simulink model "Waermepumpe"  (R2013a)
settings: Solver=ode45  StartTime=0.0  StopTime=1000  RelTol=1e-3
libraries: Thermolib x21
settings Model: Creator=admin  LastModifiedBy=studi

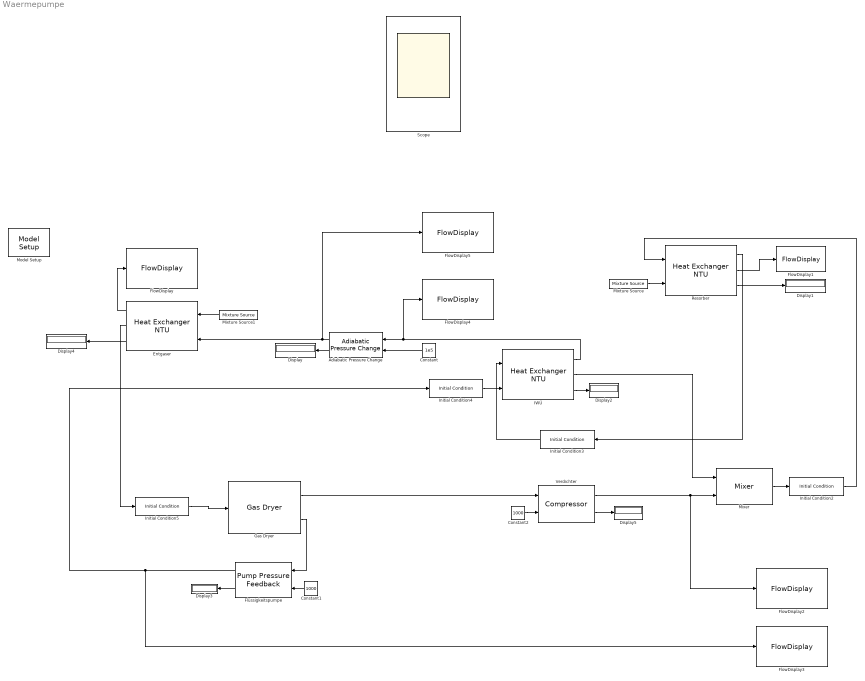
== system Waermepumpe ==
  Adiabatic Pressure Change : Thermolib/Thermodynamic State Changes/Adiabatic Pressure Change
  Constant : Constant  Value=1e5
  Constant1 : Constant  Value=1000
  Constant2 : Constant  Value=1000
  Display{,1..5} (6 alike) : Display
  Entgaser : Thermolib/Components/Heat and Mass Transfer/Heat Exchanger NTU  selection=Counter Flow  show_UA_port=off  UA_Overall=1e3  T_initial=273+25  A_env=1  T_env=273+25  k_env=0  p_loss_1=[0,1e3]  p_loss_2=[0,1e3]  thermal_mass=1*4.18e3  UA_flow1_mass1=0  UA_flow2_mass2=0  show_pf_ports=off  show_info_port=off  default_order_in_ports={'in1','in2','PFin1','PFin2'}  default_order_out_ports={'out1','out2','Qdot','PFout1','PFout2','info'}
  FlowDisplay : Thermolib/Sinks/FlowDisplay  bus_type=FlowBus  mdot=off kg/s  m_unit=mg  ndot=on mol/s  n_unit=mmol  temperature=on  T_unit=Kelvin  pressure=on  p_unit=Pa  enthalpy=off  Hdot_unit=W  H_unit=mJ  entropy=off  Sdot_unit=W/K  S_unit=mJ/K  gibbs_energy=off  Gdot_unit=W  G_unit=mJ  heat_capacity=on  Cpdot_unit=W/K  Cp_unit=mJ/K  energy_content=off  U_unit=mW/K  vapor_fraction=off  molar_fraction=off  flag=0.0921
  FlowDisplay1 : Thermolib/Sinks/FlowDisplay  bus_type=FlowBus  mdot=off kg/s  m_unit=mg  ndot=on mol/s  n_unit=mmol  temperature=on  T_unit=Kelvin  pressure=on  p_unit=Pa  enthalpy=on  Hdot_unit=W  H_unit=mJ  entropy=off  Sdot_unit=W/K  S_unit=mJ/K  gibbs_energy=off  Gdot_unit=W  G_unit=mJ  heat_capacity=off  Cpdot_unit=W/K  Cp_unit=mJ/K  energy_content=off  U_unit=mW/K  vapor_fraction=off  molar_fraction=off  flag=0.1161
  FlowDisplay2 : Thermolib/Sinks/FlowDisplay  bus_type=FlowBus  mdot=off kg/s  m_unit=mg  ndot=on mol/s  n_unit=mmol  temperature=on  T_unit=Kelvin  pressure=on  p_unit=bar  enthalpy=off  Hdot_unit=W  H_unit=mJ  entropy=off  Sdot_unit=W/K  S_unit=mJ/K  gibbs_energy=off  Gdot_unit=W  G_unit=mJ  heat_capacity=on  Cpdot_unit=W/K  Cp_unit=mJ/K  energy_content=off  U_unit=mW/K  vapor_fraction=off  molar_fraction=off  flag=0.4963
  FlowDisplay3 : Thermolib/Sinks/FlowDisplay  bus_type=FlowBus  mdot=off kg/s  m_unit=mg  ndot=on mol/s  n_unit=mmol  temperature=on  T_unit=Kelvin  pressure=on  p_unit=bar  enthalpy=off  Hdot_unit=W  H_unit=mJ  entropy=off  Sdot_unit=W/K  S_unit=mJ/K  gibbs_energy=off  Gdot_unit=W  G_unit=mJ  heat_capacity=on  Cpdot_unit=W/K  Cp_unit=mJ/K  energy_content=off  U_unit=mW/K  vapor_fraction=off  molar_fraction=off  flag=0.3209
  FlowDisplay4 : Thermolib/Sinks/FlowDisplay  bus_type=FlowBus  mdot=off kg/s  m_unit=mg  ndot=on mol/s  n_unit=mmol  temperature=on  T_unit=Kelvin  pressure=on  p_unit=bar  enthalpy=off  Hdot_unit=W  H_unit=mJ  entropy=off  Sdot_unit=W/K  S_unit=mJ/K  gibbs_energy=off  Gdot_unit=W  G_unit=mJ  heat_capacity=on  Cpdot_unit=W/K  Cp_unit=mJ/K  energy_content=off  U_unit=mW/K  vapor_fraction=off  molar_fraction=off  flag=0.5847
  FlowDisplay5 : Thermolib/Sinks/FlowDisplay  bus_type=FlowBus  mdot=off kg/s  m_unit=mg  ndot=on mol/s  n_unit=mmol  temperature=on  T_unit=Kelvin  pressure=on  p_unit=bar  enthalpy=off  Hdot_unit=W  H_unit=mJ  entropy=off  Sdot_unit=W/K  S_unit=mJ/K  gibbs_energy=off  Gdot_unit=W  G_unit=mJ  heat_capacity=on  Cpdot_unit=W/K  Cp_unit=mJ/K  energy_content=off  U_unit=mW/K  vapor_fraction=off  molar_fraction=off  flag=0.7896
  Flüssigkeitspumpe : Thermolib/Components/Hydraulic with Pressure Feedback/Pump Pressure Feedback  Mode=feed  eta_pump="[0.0 1.0;  0.8  0.8]"  RPM=[0 3000 4000 5000]  mdot=[0 8 16 24 32 34]*1e6/3600  PressureRise=[0 0 0 0 0 0 ; 13 12 10.7 8.3 3 0 ; 13 12 10.7 8.3 3 0; 13 12 10.7 8.3 3 0]*9.81e3  max_mdot=34e6/3600  p_refrence=2e5  p_Relaxation=10  show_pf_ports=off  show_info_port=off  default_order_in_ports={'in','RPM','PFin'}  default_order_out_ports={'out','P_mch','PFout','info'}
  Gas Dryer : Thermolib/Components/Heat and Mass Transfer/Gas Dryer  Abscheid_eff=[1 1 1 1 1]  ndots=[0 0.05 0.2 1 1.1]  P_Loss=[0.0,1e3]  show_pf_ports=off  show_info_port=off  default_order_in_ports={'in','PFin'}  default_order_out_ports={'out','liquid','PFout','info'}
  IWÜ : Thermolib/Components/Heat and Mass Transfer/Heat Exchanger NTU  selection=Counter Flow  show_UA_port=off  UA_Overall=1e3  T_initial=273+25  A_env=1  T_env=273+20  k_env=0  p_loss_1=[0,1e3]  p_loss_2=[0,1e3]  thermal_mass=1*4.18e3  UA_flow1_mass1=0  UA_flow2_mass2=0  show_pf_ports=off  show_info_port=off  default_order_in_ports={'in1','in2','PFin1','PFin2'}  default_order_out_ports={'out1','out2','Qdot','PFout1','PFout2','info'}
  Initial Condition2 : Thermolib/Miscellaneous/Initial Condition  disp_str=fprintf('Initial conditions:\n T = 298.15 [K]\np = 100000 [Pa]')  T=298.15 C  T_in=25  p=100000 bar  p_in=1  psi=[0 0.7 0 0 0 0 0.3]  species_local={'H2O', 'NH3'}  psi_local=[0.7 0.3]  use_fb=on  ndot=1 mol/s  ndot_in=0  switch_flow_type=1  flow_type=Molar Flow  Hdot=-215050.293043034  Sdot=101.474737141616  Gdot=-245304.985921807  Cpdot=66.5155139210582  x=[1;0.00948513258368692;1;1;1;1;0.749810260363053]  show_pf_ports=off  default_order_in_ports=off  default_order_out_ports=off
  Initial Condition3 : Thermolib/Miscellaneous/Initial Condition  disp_str=fprintf('Initial conditions:\n T = 298.15 [K]\np = 100000 [Pa]')  T=298.15 C  T_in=25  p=100000 bar  p_in=1  psi=[0 0.7 0 0 0 0 0.3]  species_local={'H2O', 'NH3'}  psi_local=[0.7 0.3]  use_fb=on  ndot=1 mol/s  ndot_in=0  switch_flow_type=1  flow_type=Molar Flow  Hdot=-215050.293043034  Sdot=101.474737141616  Gdot=-245304.985921807  Cpdot=66.5155139210582  x=[1;0.00948513258368692;1;1;1;1;0.749810260363053]  show_pf_ports=off  default_order_in_ports=off  default_order_out_ports=off
  Initial Condition4 : Thermolib/Miscellaneous/Initial Condition  disp_str=fprintf('Initial conditions:\n T = 298.15 [K]\np = 100000 [Pa]')  T=298.15 C  T_in=25  p=100000 bar  p_in=1  psi=[0 0.7 0 0 0 0 0.3]  species_local={'H2O', 'NH3'}  psi_local=[0.7 0.3]  use_fb=on  ndot=1 mol/s  ndot_in=0  switch_flow_type=1  flow_type=Molar Flow  Hdot=-215050.293043034  Sdot=101.474737141616  Gdot=-245304.985921807  Cpdot=66.5155139210582  x=[1;0.00948513258368692;1;1;1;1;0.749810260363053]  show_pf_ports=off  default_order_in_ports=off  default_order_out_ports=off
  Initial Condition5 : Thermolib/Miscellaneous/Initial Condition  disp_str=fprintf('Initial conditions:\n T = 333.15 [K]\np = 100000 [Pa]')  T=333.15 C  T_in=60  p=100000 bar  p_in=1  psi=[0 0 0 0 0 0 1]  species_local={'NH3'}  psi_local=1  use_fb=on  ndot=1 mol/s  ndot_in=0  switch_flow_type=1  flow_type=Molar Flow  Hdot=-44724.9907356956  Sdot=196.681298556579  Gdot=-110249.36534982  Cpdot=36.5745375984527  x=[0;0;0;0;0;0;1]  show_pf_ports=off  default_order_in_ports=off  default_order_out_ports=off
  Mixer : Thermolib/Components/Hydraulic/Mixer  Mode=mixer  P_Loss=[0.001,0.01e5]  p_out_method=p_out = weighted_mean(p1_in;p2_in)  default_order_in_ports={'in1','in2','ratio','PFin'}  default_order_out_ports={'out','in2 ','PFout1','PFout2','info'}  show_pf_ports=off  show_info_port=off
  Mixture Source : Thermolib/Sources/Mixture Source  disp_str=fprintf('Molar flow')  flow_type=Molar flow  switch_flow_type=1  ndot=3 mol/s  ndot_in=3  T=300 K  T_in=300  p=100000 Pa  p_in=1e+5  psi=[0 0.7 0 0 0 0 0.3]  species_local={'H2O', 'NH3'}  psi_local=[0.7 0.3]
  Mixture Source1 : Thermolib/Sources/Mixture Source  disp_str=fprintf('Molar flow')  flow_type=Molar flow  switch_flow_type=1  ndot=1.5 mol/s  ndot_in=1.5  T=300 K  T_in=300  p=100000 Pa  p_in=1e+5  psi=[0 0 0 0 0.79 0.21 0]  species_local={'N2', 'O2'}  psi_local=[0.79 0.21]
  Model Setup : Thermolib/Setup/Model Setup  starttime=10  endtime=20  loadWS=on  loadWSCommand=fc_LoadWorkspace  media_file=ChemicalMediaData.mat  constants_file=Constants.mat  species_reduced={'H2O', 'NH3', 'N2', 'O2'}  load_model_command=load ComponentData.mat  gas_eos_method=1  gas_mixing_rule=0  species_allow_liquid=[1 1 1 1]  species_allow_vapor=[1 1 1 1]  last_saved_thermolib_version=5.1.2.5490  liquid_eos_method=1  density_calculation_mode=0
  Resorber : Thermolib/Components/Heat and Mass Transfer/Heat Exchanger NTU  selection=Counter Flow  show_UA_port=off  UA_Overall=1e3  T_initial=273+25  A_env=1  T_env=273+25  k_env=0  p_loss_1=[0,1e3]  p_loss_2=[0,1e3]  thermal_mass=1*4.18e3  UA_flow1_mass1=0  UA_flow2_mass2=0  show_pf_ports=off  show_info_port=off  default_order_in_ports={'in1','in2','PFin1','PFin2'}  default_order_out_ports={'out1','out2','Qdot','PFout1','PFout2','info'}
  Scope : Scope
  Verdichter : Thermolib/Components/Hydraulic/Compressor  Mode=mechanic  tau1=1  efficiency=[100 100 100 100 100]  mass_flow=[ 1 10 15 20 30]  n_poly=1.5  max_mdot=1000  default_order_in_ports={'in','ctrl','RPM','outlet press.','P_mch ','PFin'}  default_order_out_ports={'out','P_mch','Qdot','mdot','PFout','info'}  Ref_Cond=[298 1e5]  RPM="[ 2351 2935 3518 4092  4650  5268 5870  6453]*sqrt(298)"  PR="[ 1.24 1.20 1.17 0.00 0.00 0.00 0.00 0.00 0.00; 1.40 1.39 1.38 1.34 1.32 1.29 0.00 0.00 0.00;   1.40 1.39 1.38 1.34 1.32 1.29 0.00 0.00 0.00;    1.85 1.83 1.82 1.78 1.74 1.70 1.66 0.00 0.00;    2.17 2.16 2.13 2.09 2.04 1.97 1.91 0.00 0.00;  2.5611 2.54202 2.49298 2.44727 2.36663 2.29135 0 0 0;   2.98364 2.95899 2.91164 2.86235 2.81291 0 0 0 0;  3.34342 3.30925 3.26916 3.22172 0 0 0 0 0]"  mdot="[ 0.91 1.77 2.00 0 0 0 0 0 0; 1.24 1.45 1.88 2.16 2.36 2.57 0.00 0.00 0.00;  1.66 1.82 1.96 2.13 2.31 2.60 2.79 2.96 3.10;  2.11 2.75 2.94 3.21 3.39 3.56 3.71 0.00 0.00;  2.64 3.30 3.49 3.75 3.90 4.05 4.15 0.00 0.00;  3.19797 3.82882 4.18403 4.3479 4.53375 4.63448 0 0 0; 3.7772 4.38692 4.65708 4.8777 5.01331 0 0 0 0;  4.25855 4.69137 4.91179 5.13237 0 0 0 0 0] *1e3*1.5/sqrt(298)"  eta="[ 0.60 0.60 0.55 0.00 0.00 0.00 0.00 0.00 0.00;  0.65 0.68 0.68 0.65 0.60 0.55 0.00 0.00 0.00;  0.68 0.70 0.71 0.71 0.70 0.68 0.65 0.60 0.55;   0.71 0.71 0.7 0.68 0.65 0.6 0.55 0 0;  0.71 0.71 0.7 0.68 0.65 0.6 0.55 0 0;  0.7 0.7 0.68 0.65 0.6 0.55 0 0 0; 0.68 0.68 0.65 0.6 0.55 0 0 0 0;  0.65 0.65 0.6 0.55 0 0 0 0 0]*100"  mdot_table=0  eta_table=0  PR_break=1:0.1:3  show_pf_ports=off  show_info_port=off
  wires:
  IWÜ/2 -> Mixer/1
  Gas Dryer/2 -> Flüssigkeitspumpe/1
  Flüssigkeitspumpe/1 -> FlowDisplay3/1, Initial Condition4/1
  Resorber/1 -> Initial Condition3/1
  Entgaser/2 -> Initial Condition5/1
  Mixer/1 -> Initial Condition2/1
  Adiabatic Pressure Change/1 -> FlowDisplay5/1, Entgaser/2
  Verdichter/1 -> FlowDisplay2/1, Mixer/2
  Mixture Source1/1 -> Entgaser/1
  Entgaser/1 -> FlowDisplay/1
  Adiabatic Pressure Change/2 -> Display/1
  Constant/1 -> Adiabatic Pressure Change/2
  Mixture Source/1 -> Resorber/2
  Resorber/2 -> FlowDisplay1/1
  IWÜ/1 -> FlowDisplay4/1, Adiabatic Pressure Change/1
  Resorber/3 -> Display1/1
  IWÜ/3 -> Display2/1
  Constant1/1 -> Flüssigkeitspumpe/2
  Gas Dryer/1 -> Verdichter/1
  Flüssigkeitspumpe/2 -> Display3/1
  Entgaser/3 -> Display4/1
  Constant2/1 -> Verdichter/2
  Verdichter/2 -> Display5/1
  Initial Condition2/1 -> Resorber/1
  Initial Condition3/1 -> IWÜ/1
  Initial Condition4/1 -> IWÜ/2
  Initial Condition5/1 -> Gas Dryer/1
  ? -> Scope/1
